simulink model "LPF_IMP_STEP_test"  (R2025b)
settings: Solver=VariableStepAuto  StartTime=0.0  StopTime=120  RelTol=1e-3
libraries: dspsrcs4 x3, simulink_extras x1, modelsimlib x1
settings Model: Creator=leoribeiro  LastModifiedBy=leoribeiro

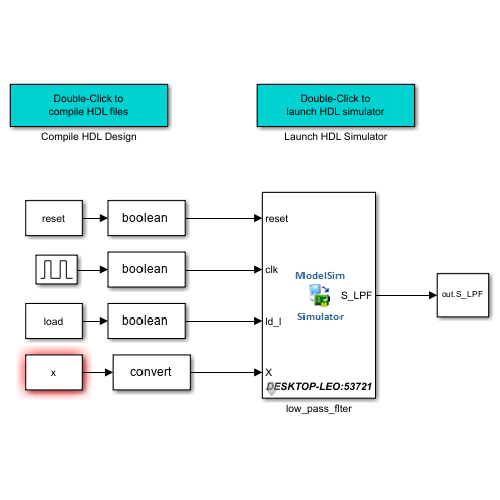
[thumbnail: Simulink's stored preview of the top-level diagram]
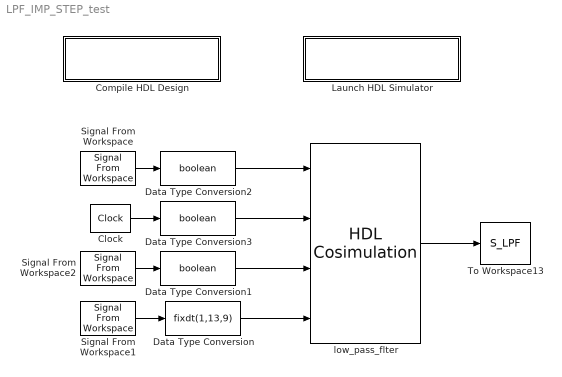
== system LPF_IMP_STEP_test ==
  Clock : simulink_extras/Flip Flops/Clock  period=1
  Compile HDL Design : Subsystem
      settings: OpenFcn=eval('compile_hdl_design_low_pass_flter');
      mask Display: disp(['Double-Click to' char(10) 'compile HDL files'])
  Data Type Conversion : DataTypeConversion  OutDataTypeStr=fixdt(1,13,9)  SaturateOnIntegerOverflow=off  RndMeth=Floor
  Data Type Conversion1 : DataTypeConversion  OutDataTypeStr=boolean  SaturateOnIntegerOverflow=off  RndMeth=Floor
  Data Type Conversion2 : DataTypeConversion  OutDataTypeStr=boolean  SaturateOnIntegerOverflow=off  RndMeth=Floor
  Data Type Conversion3 : DataTypeConversion  OutDataTypeStr=boolean  SaturateOnIntegerOverflow=off  RndMeth=Floor
  Launch HDL Simulator : Subsystem
      settings: OpenFcn=eval('launch_hdl_simulator_low_pass_flter');
      mask Display: disp(['Double-Click to' char(10) 'launch HDL simulator'])
  Signal From Workspace : dspsrcs4/Signal From Workspace  X=reset  Ts=1  nsamps=1  OutputAfterFinalValue=Setting to zero  ignoreOrWarnInputAndFrameLengths=off  OutputFrames=off
  Signal From Workspace1 : dspsrcs4/Signal From Workspace  X=x  Ts=1  nsamps=1  OutputAfterFinalValue=Setting to zero  ignoreOrWarnInputAndFrameLengths=off  OutputFrames=off
  Signal From Workspace2 : dspsrcs4/Signal From Workspace  X=load  Ts=1  nsamps=1  OutputAfterFinalValue=Setting to zero  ignoreOrWarnInputAndFrameLengths=off  OutputFrames=off
  To Workspace13 : ToWorkspace  VariableName=S_LPF  SampleTime=-1
      settings: Save2DSignal=2-D array (concatenate along first dimension)
  low_pass_flter : modelsimlib/HDL Cosimulation  PortPaths=/low_pass_flter/reset;/low_pass_flter/clk;/low_pass_flter/ld_l;/low_pass_flter/X;/low_pass_flter/S_LPF;  PortModes=[1 1 1 1 2 ]  PortTimes=[-1,-1,-1,-1,1]  PortSigns=[-1,-1,-1,-1,1,]  PortFracLengths=[0,0,0,0,9]  PortWordLengths=[-1,-1,-1,-1,16]  PortHDLWordSizes=[1,1,1,13,16]  CommLocal=on  CommSharedMemory=off  CommPortNumber=53721  CommShowInfo=on  ClockModes=[]  ClockTimes=[]  TclPreSimCommand="puts \"Running Simulink Cosimulation block.\""  TclPostSimCommand="puts \"done\";"  TimingMode=ns  TimingScaleFactor=100  idxCellArray={'UNUSED_VAR'}  CosimBypass=Full Simulation  AllowDirectFeedthrough=on  ProductName=EDA Simulator Link MQ  RunAutoTimescale=off  HdlClocks=0  PreRunTime=0  PreRunTimeUnit=ns
  wires:
  Signal From Workspace1/1 -> Data Type Conversion/1
  Data Type Conversion/1 -> low_pass_flter/4
  Data Type Conversion1/1 -> low_pass_flter/3
  Signal From Workspace/1 -> Data Type Conversion2/1
  Data Type Conversion2/1 -> low_pass_flter/1
  Signal From Workspace2/1 -> Data Type Conversion1/1
  Data Type Conversion3/1 -> low_pass_flter/2
  Clock/1 -> Data Type Conversion3/1
  low_pass_flter/1 -> To Workspace13/1

== system LPF_IMP_STEP_test/Compile HDL Design ==

== system LPF_IMP_STEP_test/Launch HDL Simulator ==
